simulink model "Pitch1doF_NL"  (R2019b)
settings: Solver=VariableStepAuto  StartTime=0.0  StopTime=10.0  RelTol=1e-3
undefined symbols (not defined in the file): Dm, Dt, g, J_eq, K_pitch, Mb
settings Model: Creator=lbend  LastModifiedBy=lbend

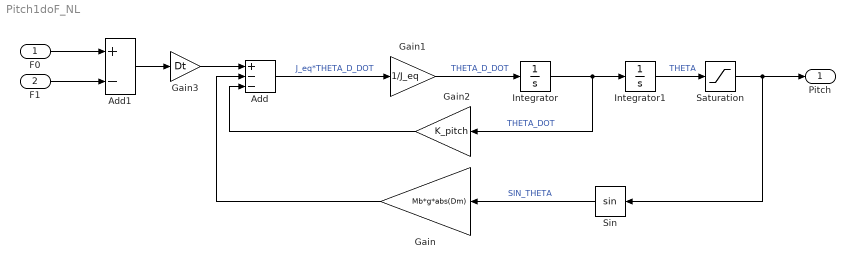
== system Pitch1doF_NL ==
  F0 : Inport
  "F1 " : Inport  Port=2
  Add : Sum  Inputs=+--
  Add1 : Sum  Inputs=+-
  Gain : Gain  Gain=Mb*g*abs(Dm)
  Gain1 : Gain  Gain=1/J_eq
  Gain2 : Gain  Gain=K_pitch
  Gain3 : Gain  Gain=Dt
  Integrator : Integrator
  Integrator1 : Integrator
  Saturation : Saturate  UpperLimit=0.93  LowerLimit=-0.93
  Sin : Trigonometry
  Pitch : Outport
  wires:
  Add1/1 -> Gain3/1
  Gain1/1 -> Integrator/1  "THETA_D_DOT"
  Gain3/1 -> Add/1
  Add/1 -> Gain1/1  "J_eq*THETA_D_DOT"
  F0/1 -> Add1/1
  Integrator1/1 -> Saturation/1  "THETA"
  Gain2/1 -> Add/3
  "F1 "/1 -> Add1/2
  Gain/1 -> Add/2
  Integrator/1 -> Gain2/1, Integrator1/1  "THETA_DOT"
  Sin/1 -> Gain/1  "SIN_THETA"
  Saturation/1 -> Sin/1, Pitch/1
